simulink model "MATMPC_SIMULINK"  (R2022b)
settings: Solver=FixedStepAuto  StartTime=0.0  StopTime=4.0  RelTol=1e-3
values from neighbouring files (symbols this model uses):
  lb = 0    [Initialization_Simulink.m]
  lbu = -inf(nu,1)    [InitData.m]    (also in Initialization_Simulink.m = repmat(lbu,1,N))
  lbx = 0    [Initialization_Simulink.m]
  para = repmat(para0,1,N+1)    [InitData.m]    (also in Initialization_Simulink.m)
  Ts = settings.Ts_st    [Initialization_Simulink.m]    (also in Simulation.m)
  ub = 0    [Initialization_Simulink.m]
  ubu = inf(nu,1)    [InitData.m]    (also in Initialization_Simulink.m = repmat(ubu,1,N))
  ubx = 0    [Initialization_Simulink.m]
  W = repmat([10 10 0.1 0.1 0.01]',1,N)    [Initialization_Simulink.m]
  WN = W(1:nyN,1)    [Initialization_Simulink.m]
  x0 = [0;pi;0;0]    [Initialization_Simulink.m]
  z0 = 0    [Initialization_Simulink.m]
undefined symbols (not defined in the file or in its folder): opt, settings
settings Model: Creator=chen  LastModifiedBy=beniamino
settings SolverCC: AlgebraicLoopSolver=TrustRegion
settings DataIOCC: ReturnWorkspaceOutputs=off
settings DebuggingCC: UnconnectedInputMsg=warning  UnconnectedOutputMsg=warning  UnconnectedLineMsg=warning  SFMachineParentedDataDiag=warning  ArithmeticOperatorsInVariantConditions=warning
settings ModelReferenceCC: EnableRefExpFcnMdlSchedulingChecks=on
settings SFSimCC: SimUseLocalCustomCode=off  CustomCodeUndefinedFunction=UseInterfaceOnly
settings RTWCC: RTWUseLocalCustomCode=off  CheckMdlBeforeBuild=Error

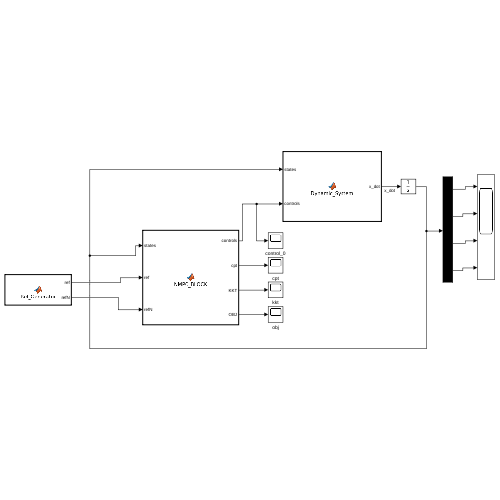
[thumbnail: Simulink's stored preview of the top-level diagram]
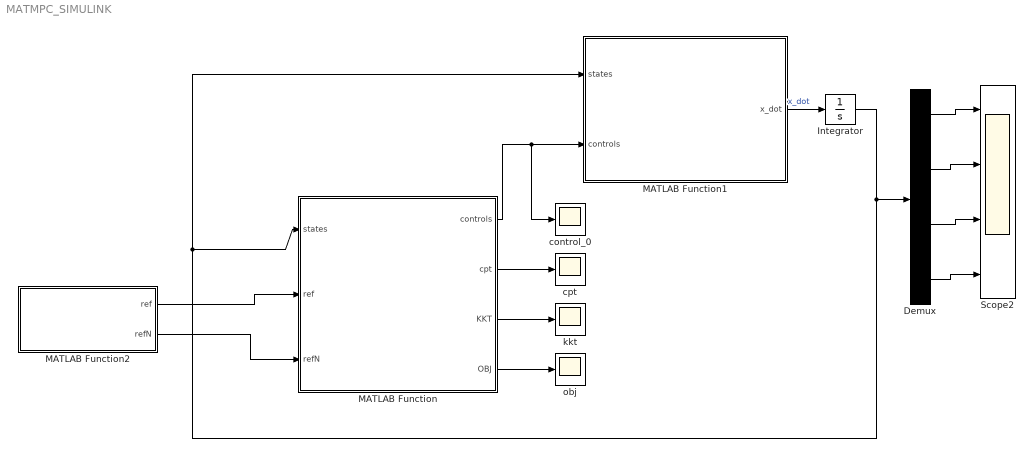
== system MATMPC_SIMULINK ==
  Demux : Demux
  Integrator : Integrator  InitialCondition=x0
  MATLAB Function : MATLAB Function  TreatAsAtomicUnit=on  SystemSampleTime=Ts
  MATLAB Function1 : MATLAB Function  TreatAsAtomicUnit=on
  MATLAB Function2 : MATLAB Function  TreatAsAtomicUnit=on
  Scope2 : Scope  NumInputPorts=4
  control_0 : Scope
  cpt : Scope
  kkt : Scope
  obj : Scope
  wires:
  MATLAB Function/1(controls) -> control_0/1, MATLAB Function1/2(controls)
  MATLAB Function1/1(x_dot) -> Integrator/1  "x_dot"
  Integrator/1 -> Demux/1, MATLAB Function/1(states), MATLAB Function1/1(states)
  Demux/1 -> Scope2/1
  Demux/2 -> Scope2/2
  Demux/3 -> Scope2/3
  Demux/4 -> Scope2/4
  MATLAB Function/2(cpt) -> cpt/1
  MATLAB Function/4(OBJ) -> obj/1
  MATLAB Function/3(KKT) -> kkt/1
  MATLAB Function2/1(ref) -> MATLAB Function/2(ref)
  MATLAB Function2/2(refN) -> MATLAB Function/3(refN)

== matlab function MATMPC_SIMULINK/MATLAB Function2 ==
  data: ref output; settings parameter; refN output
function [ref,refN] = Ref_Generator(settings)

ref=zeros(settings.ny,settings.N);
refN=zeros(settings.nyN,1);

%     ref = repmat([1.4, 0, 0]',1,settings.N);
%     refN = 1.4;

== matlab function MATMPC_SIMULINK/MATLAB Function1 ==
  data: states input size=nx; x_dot output size=nx; controls input size=nu
function x_dot  = Dynamic_System(states,controls)

M = 1; 
m = 0.1;
l = 0.8; 
g = 9.81;

p=states(1);
theta=states(2);
v=states(3);
omega=states(4);  
u=controls(1);

a=-m*l*sin(theta)*omega^2+m*g*cos(theta)*sin(theta)+u;
b=-m*l*cos(theta)*sin(theta)*omega^2+u*cos(theta)+(M+m)*g*sin(theta);
c=M+m-m*(cos(theta))^2;

x_dot = [v;omega;a/c;b/(l*c)];

return

== matlab function MATMPC_SIMULINK/MATLAB Function ==
  settings: updateMethod=DISCRETE
  data: states input size=nx; settings parameter; opt parameter; lb parameter; ub parameter; lbx parameter; ubx parameter; lbu parameter; ubu parameter; W parameter; WN parameter; para parameter; ref input size=[ny N]; refN input size=nyN; z0 parameter; controls output size=nu; cpt output size=1; KKT output; OBJ output
function [controls, cpt, KKT, OBJ] = NMPC_BLOCK(states, settings, opt, lb, ub, lbx, ubx, lbu, ubu, W, WN, para, ref, refN, z0)

%% everything should has a fixed size
coder.extrinsic('mpc_nmpcsolver_simulink');  
coder.extrinsic('InitData');  
coder.extrinsic('InitMemory');  
coder.extrinsic('evalin');
coder.extrinsic('assignin');

%%

persistent x u z lambda mu mu_x mu_u;
persistent input mem;

if isempty(input)  
    
    nx = settings.nx;        % No. of differential states
    nu = settings.nu;        % No. of controls
    nz = settings.nz;        % No. of algebraic states
    ny = settings.ny;        % No. of outputs (references)    
    nyN= settings.nyN;       % No. of outputs at terminal stage 
    np = settings.np;        % No. of parameters (on-line data)
    nc = settings.nc;        % No. of constraints
    ncN = settings.ncN;      % No. of constraints at terminal stage
    nbu = settings.nbu;      % No. of control bounds
    nbx = settings.nbx;      % No. of state bounds
    nbu_idx = settings.nbu_idx; % Index of control bounds
    nbx_idx = settings.nbx_idx; % Index of state bounds
    N = settings.N;
    N2 = settings.N2;
    r = settings.r;
        
    input.x0=states;
    
    x=repmat(states,1,N+1);
    input.x=x;
    
    u=zeros(nu,N);
    input.u=u;
    
    z=repmat(z0,1,N);
    input.z=z;
    
    lambda = zeros(nx,N+1);
    input.lambda= lambda;
    
    if N*nc+ncN > 0
        mu = zeros(N*nc+ncN,1);
    else
        mu = 0;
    end
    input.mu= mu;
    
    mu_u = zeros(N*nu,1);
    input.mu_u= mu_u;
    
    if N*nbx > 0
        mu_x = zeros(N*nbx,1);
    else
        mu_x = 0;
    end
    input.mu_x = mu_x;
    
    input.W=W;
    input.WN=WN;
    input.od = para;
    
    input.lb = lb;
    input.ub = ub;
    input.lbx = lbx;
    input.ubx = ubx;
    input.lbu = lbu;
    input.ubu = ubu;
      
    input.y = ref;
    input.yN = refN;
    
    mem = InitMemory(settings, opt, input);
        
else

    input.x=x; 
    input.u=u;
    input.z=z;
    input.lambda=lambda;   
    input.mu=mu;
    input.mu_x=mu_x;
    input.mu_u=mu_u;
    
    input.od = para;
    input.y = ref;
    input.yN = refN;
    
end

%%
cpt = 0;
KKT = 0;
OBJ = 0;
input.x0 = states;
[input,mem,cpt,KKT,OBJ] = mpc_nmpcsolver_simulink(input, settings, mem, opt);
controls = input.u(1,1);

%% shifting
switch opt.shifting
    case 'yes'
        x=[input.x(:,2:end),input.x(:,end)];  
        u=[input.u(:,2:end),input.u(:,end)]; 
        z=[input.z(:,2:end),input.z(:,end)]; 
        lambda=[input.lambda(:,2:end),input.lambda(:,end)];
        if (settings.N*settings.nc+settings.ncN) >0
            mu(1:end-settings.ncN+1)=input.mu(settings.nc+1:settings.N*settings.nc+settings.ncN,1);
            mu(settings.N*settings.nc+1:end)=input.mu(settings.N*settings.nc+settings.ncN-settings.nc+1:settings.N*settings.nc+settings.ncN,1);
        else
            mu=0;
        end
        mu_x=[input.mu_x(2:end,1);input.mu_x(end,1)];
        mu_u=[input.mu_u(2:end,1);input.mu_u(end,1)];
   case 'no'
        x=input.x;
        u=input.u;
        z=input.z;
        lambda=input.lambda;
        mu=input.mu;
        mu_x=input.mu_x;
        mu_u=input.mu_u;
end

return
